simulink model "lqr_hovering_ENU_linear"  (R2017a)
settings: Solver=ode4  StartTime=0.0  StopTime=30  FixedStep=Ts  RelTol=1e-3  EnableMultiTasking=on
values from neighbouring files (symbols this model uses):
  Ac = [0 0 0  1 0 0   0  0  0  0 0 0 ... (first row only)    [lqr_hovering_ENU_synthesis.m]
  Bc = [zeros(3,4) ... (first row only)    [lqr_hovering_ENU_synthesis.m]
  Cc = [eye(3) zeros(3,9) ... (first row only)    [lqr_hovering_ENU_synthesis.m]
  Ki_lqr = [0 0 0.1 0 0 -0.1 0 0 8.66025403784 0 0 0 ... (16 elements, 4x4)]    [K_lqr_hovering_ENU.mat]    (also in lqr_hovering_ENU_synthesis.m = -K(:,13:end))
  Kx_lqr = [0 0 0.263619393691 0 0 -0.257300038922 0 0 13.5913339138 0 0 0 ... (48 elements, 4x12)]    [K_lqr_hovering_ENU.mat]    (also in lqr_hovering_ENU_synthesis.m = K(:,1:12))
undefined symbols (not defined in the file or in its folder): B_ENU_inv, gra, KT, mass
settings Model: Creator=dtnguyen  LastModifiedBy=ducnguyen
settings DataIOCC: LimitDataPoints=on  SaveFormat=Array
settings OptimizationCC: DefaultParameterBehavior=Inlined  UseFloatMulNetSlope=on  InlineInvariantSignals=on  EfficientFloat2IntCast=on  LifeSpan=inf
settings DebuggingCC: SFUnexpectedBacktrackingDiag=warning  SFNoUnconditionalDefaultTransitionDiag=warning  SFExecutionAtInitializationDiag=none
settings HardwareCC: ProdBitPerPointer=32  ProdBitPerSizeT=32  ProdBitPerPtrDiffT=32  ProdLargestAtomicFloat=None  ProdIntDivRoundTo=Undefined  ProdEndianess=Unspecified  ProdWordSize=32  ProdHWDeviceType=32-bit Generic
settings ModelReferenceCC: PropagateSignalLabelsOutOfModel=off
settings RTWCC: GenerateReport=on  Toolchain=Catkin  BuildConfiguration=Faster Runs  LaunchReport=on  TargetLang=C++  CheckMdlBeforeBuild=Warning
settings GRTTargetCC: TargetLangStandard=C++03 (ISO)  GeneratePreprocessorConditionals=Disable all  MatFileLogging=off  MultiInstanceERTCode=on  CodeInterfacePackaging=C++ class  SupportNonFinite=off
settings ConfigComp: CovMetricSettings=dw  CovHtmlReporting=on  CovSaveCumulativeToWorkspaceVar=on  CovSaveSingleToWorkspaceVar=on  CovExternalEMLEnable=off

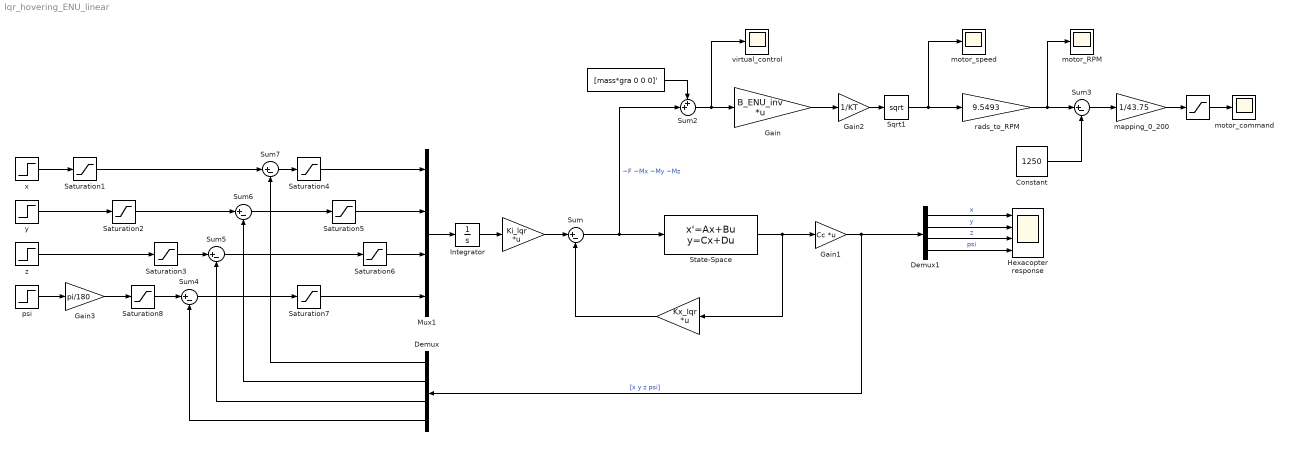
== system lqr_hovering_ENU_linear ==
  " " : Gain  Gain=Ki_lqr  Multiplication=Matrix(K*u)
  "  " : Saturate  UpperLimit=200  LowerLimit=0
  "              " : Constant  Value=[mass*gra 0 0 0]'
  "                   " : Gain  Gain=Kx_lqr  Multiplication=Matrix(K*u)
  Constant : Constant  Value=1250  VectorParams1D=off  SampleTime=-1
  Demux : Demux
  Demux1 : Demux
  Gain : Gain  Gain=B_ENU_inv  Multiplication=Matrix(K*u)
  Gain1 : Gain  Gain=Cc  Multiplication=Matrix(K*u)
  Gain2 : Gain  Gain=1/KT
  Gain3 : Gain  Gain=pi/180
  Hexacopter response : Scope  NumInputPorts=4
  Integrator : Integrator  InitialCondition=[0 0 0 0]'
  Mux1 : Mux
  Saturation1 : Saturate  UpperLimit=2  LowerLimit=-2
  Saturation2 : Saturate  UpperLimit=2  LowerLimit=-2
  Saturation3 : Saturate  UpperLimit=1.75  LowerLimit=0
  Saturation4 : Saturate  UpperLimit=1  LowerLimit=-1
  Saturation5 : Saturate  UpperLimit=1  LowerLimit=-1
  Saturation6 : Saturate
  Saturation7 : Saturate  UpperLimit=pi/4  LowerLimit=-pi/4
  Saturation8 : Saturate  UpperLimit=2*pi  LowerLimit=-2*pi
  Sqrt1 : Sqrt  SaturateOnIntegerOverflow=on
  State-Space : StateSpace  A=Ac  B=Bc  C=eye(12)  D=zeros(12,4)  X0=0
  Sum{,3..7} (6 alike) : Sum  Inputs=|+-
  Sum2 : Sum  Inputs=++|
  mapping_0_200 : Gain  Gain=1/43.75
  motor_RPM : Scope
  motor_command : Scope
  motor_speed : Scope
  psi : Step  Time=15  After=90  SampleTime=0
  rads_to_RPM : Gain  Gain=9.5493
  virtual_control : Scope
  x : Step  Time=5  SampleTime=0
  y : Step  Time=10  SampleTime=0
  z : Step  Time=0  SampleTime=0
  wires:
  Sum/1 -> State-Space/1, Sum2/2  "~F ~Mx ~My ~Mz"
  "                   "/1 -> Sum/2
  Integrator/1 -> " "/1
  " "/1 -> Sum/1
  Demux1/2 -> Hexacopter response/2  "y"
  Demux1/1 -> Hexacopter response/1  "x"
  Demux1/3 -> Hexacopter response/3  "z"
  z/1 -> Saturation3/1
  x/1 -> Saturation1/1
  y/1 -> Saturation2/1
  Mux1/1 -> Integrator/1
  State-Space/1 -> Gain1/1, "                   "/1
  Gain1/1 -> Demux1/1, Demux/1  "[x y z psi]"
  Sum2/1 -> virtual_control/1, Gain/1
  Gain2/1 -> Sqrt1/1
  rads_to_RPM/1 -> Sum3/1, motor_RPM/1
  Constant/1 -> Sum3/2
  Sum3/1 -> mapping_0_200/1
  Demux1/4 -> Hexacopter response/4  "psi"
  Gain/1 -> Gain2/1
  Saturation1/1 -> Sum7/1
  Saturation2/1 -> Sum6/1
  Saturation3/1 -> Sum5/1
  psi/1 -> Gain3/1
  Gain3/1 -> Saturation8/1
  Demux/1 -> Sum7/2
  Demux/2 -> Sum6/2
  Demux/3 -> Sum5/2
  Demux/4 -> Sum4/2
  Sum7/1 -> Saturation4/1
  Saturation4/1 -> Mux1/1
  Sum6/1 -> Saturation5/1
  Saturation5/1 -> Mux1/2
  Sum4/1 -> Saturation7/1
  Sqrt1/1 -> rads_to_RPM/1, motor_speed/1
  Sum5/1 -> Saturation6/1
  Saturation6/1 -> Mux1/3
  Saturation7/1 -> Mux1/4
  Saturation8/1 -> Sum4/1
  "              "/1 -> Sum2/1
  mapping_0_200/1 -> "  "/1
  "  "/1 -> motor_command/1
